simulink model "met_Lap_1_31"  (R2020b)
settings: Solver=VariableStepAuto  StartTime=0.0  StopTime=10.0  RelTol=1e-3
undefined symbols (not defined in the file): b, c, d, x0
settings Model: Creator=48576  LastModifiedBy=48576

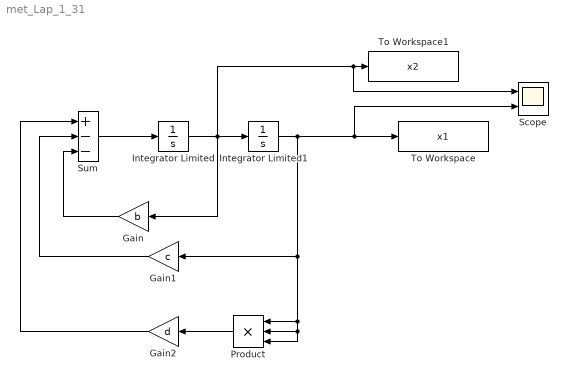
== system met_Lap_1_31 ==
  Gain : Gain  Gain=b
  Gain1 : Gain  Gain=c
  Gain2 : Gain  Gain=d
  Integrator Limited : Integrator  InitialCondition=x0(1)  LimitOutput=on  UpperSaturationLimit=2  LowerSaturationLimit=-2
  Integrator Limited1 : Integrator  InitialCondition=x0(2)  LimitOutput=on  UpperSaturationLimit=2  LowerSaturationLimit=-2
  Product : Product  Inputs=3
  Scope : Scope  NumInputPorts=2
  Sum : Sum  Inputs=+--
  To Workspace : ToWorkspace  VariableName=x1  SampleTime=-1
  To Workspace1 : ToWorkspace  VariableName=x2  SampleTime=-1
  wires:
  Sum/1 -> Integrator Limited/1
  Integrator Limited/1 -> Integrator Limited1/1, Scope/1, To Workspace1/1, Gain/1
  Gain/1 -> Sum/3
  Integrator Limited1/1 -> Scope/2, To Workspace/1, Product/1, Product/2, Product/3, Gain1/1
  Gain1/1 -> Sum/2
  Product/1 -> Gain2/1
  Gain2/1 -> Sum/1
